simulink model "HSPPreview"  (R2014b)
settings: Solver=ode3  StartTime=0.0  StopTime=10.0  FixedStep=1e-3  RelTol=1e-3
settings Model: Creator=Hyowinner  LastModifiedBy=Hyowinner
settings OptimizationCC: InlineParams=on  OptimizeModelRefInitCode=on  LifeSpan=1
settings RTWCC: SystemTargetFile=ert.tlc  TemplateMakefile=ert_default_tmf  Description=Embedded Coder  GenerateReport=on  ProcessScript=ert_make_rtw_hook  IncludeHyperlinkInReport=on  LaunchReport=on
settings CodeAppCC: IgnoreCustomStorageClasses=off
settings ERTTargetCC: GenerateSampleERTMain=on  InlinedParameterPlacement=NonHierarchical  ERTCustomFileTemplate=example_file_process.tlc

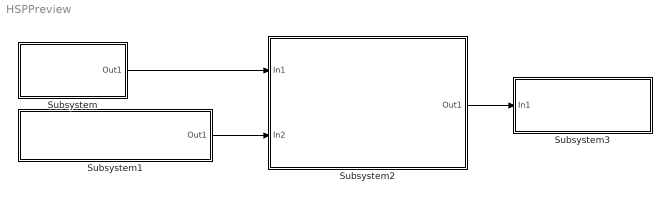
== system HSPPreview ==
  Subsystem : Subsystem
      mask Display: disp('目标芯片手册');
  Subsystem1 : Subsystem
      mask Display: disp('驱动代码集(寄存器级，应用API级等)');
  Subsystem2 : Subsystem
      mask Display: disp('C mex S Function|M script|TLC script')
  Subsystem3 : Subsystem
      mask Display: disp('Hardware Support Package');
  wires:
  Subsystem/1(Out1) -> Subsystem2/1(In1)
  Subsystem1/1(Out1) -> Subsystem2/2(In2)
  Subsystem2/1(Out1) -> Subsystem3/1(In1)

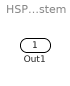
== system HSPPreview/Subsystem ==
  Out1 : Outport

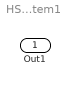
== system HSPPreview/Subsystem1 ==
  Out1 : Outport

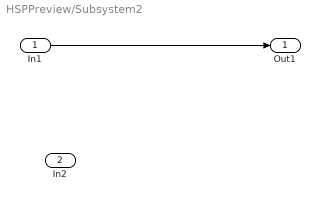
== system HSPPreview/Subsystem2 ==
  In1 : Inport
  In2 : Inport  Port=2
  Out1 : Outport
  wires:
  In1/1 -> Out1/1

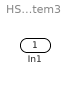
== system HSPPreview/Subsystem3 ==
  In1 : Inport
